simulink model "lab2part3"  (R2020b)
settings: Solver=VariableStepAuto  StartTime=0.0  StopTime=2.0  RelTol=1e-3
libraries: simulink x1
settings Model: Creator=Nikita  LastModifiedBy=Nikita

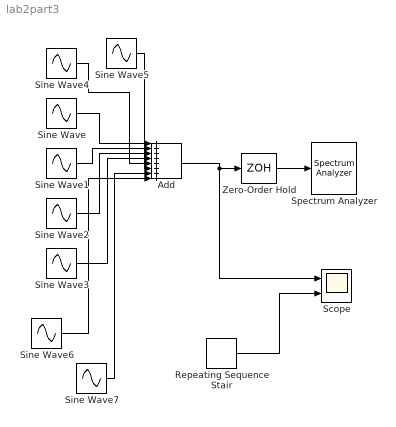
== system lab2part3 ==
  Add : Sum  Inputs=++++++++
  Repeating Sequence Stair : simulink/Sources/Repeating Sequence Stair  OutValues=[1 -1].'  tsamp=1/64  OutMin=[]  OutMax=[]  OutDataTypeStr=double  OutputDataTypeScalingMode=double  OutDataType=fixdt(0,8)  ConRadixGroup=Best Precision: Vector-wise  OutScaling=2^-12
  Scope : Scope  NumInputPorts=2
  Sine Wave : Sin  Amplitude=4/(pi*1)  Frequency=64*pi  SampleTime=0
  Sine Wave1 : Sin  Amplitude=4/(pi*3)  Frequency=192*pi  SampleTime=0
  Sine Wave2 : Sin  Amplitude=4/(pi*5)  Frequency=320*pi  SampleTime=0
  Sine Wave3 : Sin  Amplitude=4/(pi*7)  Frequency=448*pi  SampleTime=0
  Sine Wave4 : Sin  Amplitude=4/(pi*11)  Frequency=704*pi  SampleTime=0
  Sine Wave5 : Sin  Amplitude=4/(pi*9)  Frequency=576*pi  SampleTime=0
  Sine Wave6 : Sin  Amplitude=4/(pi*13)  Frequency=64*pi*13  SampleTime=0
  Sine Wave7 : Sin  Amplitude=4/(pi*15)  Frequency=64*pi*15  SampleTime=0
  Spectrum Analyzer : SpectrumAnalyzer
  Zero-Order Hold : ZeroOrderHold  SampleTime=2^-10
  wires:
  Repeating Sequence Stair/1 -> Scope/2
  Zero-Order Hold/1 -> Spectrum Analyzer/1
  Add/1 -> Scope/1, Zero-Order Hold/1
  Sine Wave3/1 -> Add/4
  Sine Wave2/1 -> Add/3
  Sine Wave1/1 -> Add/2
  Sine Wave/1 -> Add/1
  Sine Wave6/1 -> Add/8
  Sine Wave7/1 -> Add/7
  Sine Wave5/1 -> Add/6
  Sine Wave4/1 -> Add/5
